simulink model "Phase1_Mark2"  (R2024b)
settings: Solver=ode23tb  StartTime=0.0  StopTime=inf  FixedStep=.001  RelTol=1e-1
model workspace (MAT data in the model file):
  A_mu = 10
  B_reff = 8.386
  CONVERTER_DATA = [0 0.1 0.2 0.3 0.4 0.5 0.6 0.7 0.8 0.81 0.82 0.83 ... (63 elements, 21x3)]
  Cps = 2
  Cz = 7766.25
  DOWN_TABLE = [0 0 0 0 0 0 5 5 7.5 7.5 15 15 ... (30 elements, 6x5)]
  DOWN_TH_BP = [0 5 40 50 90 100]
  D_reff = 0.25826
  EMAP = [-40 215 245 264 264 267 267 267 267 267 -44 117 ... (110 elements, 10x11)]
  F0z = [6086.4 4324.8]
  F_reff = 0.07394
  F_zmax = 10000
  F_zmin = 100
  F_zo = 4000
  Kz = 48000
  MF : object (value not decoded)
  NCyl = 6
  NE_VEC = [800 1200 1600 2000 2400 2800 3200 3600 4000 4400 4800]
  Pstd = 101325
  Rair = 287
  SUS : object (value not decoded)
  TH_VEC = [0; 20; 30; 40; 50; 60; 70; 80; 90; 100]
  TWAITdn = 1.25
  TWAITup = 0.1
  Tin = [1 2 3 4 5 6 7 8 9 10 2 2 ... (20 elements, 10x2)]
  Tstd = 293.15
  UP_TABLE = [7.5 7.5 15 25 40 40 25 25 35 45 70 80 ... (30 elements, 6x5)]
  UP_TH_BP = [0 25 35 50 90 100]
  VEH : object (value not decoded)
  V_o = 16.7
  V_xlow = 1
  Vd = 0.00346
  WH : object (value not decoded)
  a = 1.515
  alpha_max = 1.5
  alpha_min = -1.5
  b = 1.504
  c_zo = 209651
  epsilon = 0.1
  f_air = [0 0 0 0 0 0 0 0 0 0 0 0 ... (256 elements, 16x16)]
  f_co = [0 0 0 0 0 0 0 0 0 0 0 0 ... (256 elements, 16x16)]
  f_co2 = [0 0 0 0 0 0 0 0 0 0 0 0 ... (256 elements, 16x16)]
  f_eff = [352.135682859 352.135682859 320.724378192 303.655312657 295.930136708 291.240087194 291.240271258 291.240312459 291.240275452 291.240198499 291.240100781 291.240018769 ... (256 elements, 16x16)]
  f_fuel = [0 0 0 0 0 0 0 0 0 0 0 0 ... (256 elements, 16x16)]
  f_hc = [0 0 0 0 0 0 0 0 0 0 0 0 ... (256 elements, 16x16)]
  f_nox = [0 0 0 0 0 0 0 0 0 0 0 0 ... (256 elements, 16x16)]
  f_pm = [0 0 0 0 0 0 0 0 0 0 0 0 ... (256 elements, 16x16)]
  f_susp_axl_bp = [1 2]
  f_susp_dz_bp = [-4 -0.14 -0.13 -0.12 -0.11 -0.1 -0.09 -0.08 -0.07 -0.06 -0.05 -0.04 ... (31 elements, 1x31)]
  f_susp_dzdot_bp = [-4 -0.14 -0.13 -0.12 -0.11 -0.1 -0.09 -0.08 -0.07 -0.06 -0.05 -0.04 ... (31 elements, 1x31)]
  f_susp_fmz = [-213379.591456 -28099.591456 -27619.591456 -27139.591456 -26659.591456 -26179.591456 -25699.591456 -25219.591456 -24739.591456 -24259.591456 -23779.591456 -23299.591456 ... (468968 elements, 31x31x61x2x4)]
  f_susp_geom = [-0.832564012244 0.043269987756 0.045538987756 0.047807987756 0.050076987756 0.052345987756 0.054614987756 0.056883987756 0.059152987756 0.061421987756 0.063690987756 0.065959987756 ... (11346 elements, 31x61x2x3)]
  f_susp_strgdelta_bp = [-0.523598775598 -0.506145483078 -0.488692190558 -0.471238898038 -0.453785605519 -0.436332312999 -0.418879020479 -0.401425727959 -0.383972435439 -0.366519142919 -0.349065850399 -0.331612557879 ... (61 elements, 1x61)]
  f_tbrake = [0 76.8593923996 105.140482948 131.533638111 157.926793274 176.658631717 176.65727296 176.656856686 176.656879077 176.657093756 176.657404516 176.65772406 ... (256 elements, 16x16)]
  f_tbrake_n_bpt = [0 649.519052838 912.419621844 1175.32019085 1438.22075986 1701.12132886 1964.02189787 2226.92246687 2489.82303588 2752.72360489 3015.62417389 3278.5247429 ... (16 elements, 1x16)]
  f_tbrake_t_bpt = [0 34.6410161514 61.0341713143 87.4273264773 113.82048164 140.213636803 166.606791966 192.999947129 219.393102292 245.786257455 272.179412618 298.572567781 ... (16 elements, 1x16)]
  f_texh = [766.752464599 766.752464599 786.17542386 801.679939032 884.591982581 910.574397722 910.571871054 910.570774534 910.570601632 910.570821151 910.571247242 910.571639815 ... (256 elements, 16x16)]
  f_twc_eff_co = [0.17 0.25 0.45 0.99 0.99 0.99 0.99]
  f_twc_eff_hc = [0.21 0.375 0.75 0.98 0.98 0.98 0.98]
  f_twc_eff_lam = [0.909090909 0.944055944 0.979020979 1 1.013986014 1.048951049 1.083916084]
  f_twc_eff_nox = [0.98 0.98 0.98 0.97 0.05 0.02 0]
  h = 0.134
  k_z = 50
  kappa_max = 1.5
  kappa_min = -1.5
  lam_Cx = 1
  lam_Cy = 1
  lam_Cz = 1
  lam_Ex = 1
  lam_Ey = 1
  lam_F_zo = 1
  lam_Hx = 1
  lam_Hy = 1
  lam_Kxkappa = 1
  lam_Kyalpha = 1
  lam_Kygamma = 1
  lam_Kzgamma = 1
  lam_Mr = 1
  lam_Mx = 1
  lam_My = 1
  lam_S = 1
  lam_VMx = 1
  lam_Vx = 1
  lam_Vy = 1
  lam_Vykappa = 1
  lam_muV = 0
  lam_mux = 1
  lam_muy = 1
  lam_t = 1
  lam_xalpha = 1
  lam_ykappa = 1
  numWheel = 4
  p_Cx1 = 1.579
  p_Cy1 = 1.3332
  p_Dx1 = 1.0422
  p_Dx2 = -0.08285
  p_Dx3 = 0
  p_Dy1 = 0.8784
  p_Dy2 = -0.06445
  p_Dy3 = 0
  p_Ex1 = 0.11185
  p_Ex2 = 0.3127
  p_Ex3 = 0
  p_Ex4 = 0.001603
  p_Ey1 = -0.8227
  p_Ey2 = -0.6062
  p_Ey3 = 0.09825
  p_Ey4 = -6.546
  p_Ey5 = 0
  p_Fz1 = 0.7098
  p_Hx1 = 0.00021585
  p_Hx2 = 0.0011538
  p_Hy1 = -0.0018043
  p_Hy2 = 0.003518
  p_Kx1 = 21.69
  p_Kx2 = 13.774
  p_Kx3 = -0.4119
  p_Ky1 = -15.314
  p_Ky2 = 1.7044
  p_Ky3 = 0.36986
  p_Ky4 = 1.9896
  p_Ky5 = 0
  p_Ky6 = -0.9004
  p_Ky7 = -0.2328
  p_Vx1 = 1.5973e-05
  p_Vx2 = 0.0001043
  p_Vy1 = -0.006642
  p_Vy2 = 0.03597
  p_Vy3 = -0.1621
  p_Vy4 = -0.4908
  p_pmx1 = 0
  p_px1 = -0.3489
  p_px2 = 0.382
  p_px3 = -0.09634
  p_px4 = 0.06447
  p_py1 = -0.6249
  p_py2 = -0.06535
  p_py3 = -0.1668
  p_py4 = 0.2834
  p_py5 = 0
  path : object (value not decoded)
  pio = 220000
  q_Fcx = 0
  q_Fz2 = 15.4
  q_Fzy = 0
  q_reo = 0.9974
  q_sx1 = -0.007764
  q_sx10 = 0.2824
  q_sx11 = 5.349
  q_sx12 = 0
  q_sx13 = 0
  q_sx14 = 0
  q_sx2 = 1.1915
  q_sx3 = 0.013948
  q_sx4 = 4.912
  q_sx5 = 1.02
  q_sx6 = 22.83
  q_sx7 = 0.7104
  q_sx8 = -0.023393
  q_sx9 = 0.6581
  q_sy1 = 0.00702
  q_sy2 = 0
  q_sy3 = 0.001515
  q_sy4 = 8.514e-05
  q_sy5 = 0
  q_sy6 = 0
  q_sy7 = 0.9008
  q_sy8 = -0.4089
  q_v1 = 0.0007742
  q_v2 = 0.04667
  r_Bx1 = 12.531
  r_Bx2 = 9.532
  r_Bx3 = 0
  r_By1 = 10.615
  r_By2 = 7.705
  r_By3 = 3.433e-06
  r_By4 = 0
  r_Cx1 = 1.019
  r_Cy1 = 1.0585
  r_Ex1 = -0.4487
  r_Ex2 = -0.4726
  r_Ey1 = 0.3132
  r_Ey2 = 7.63e-06
  r_Hx1 = 0.0002374
  r_Hy1 = 0.011646
  r_Hy2 = 7.63e-06
  r_Vy1 = 0.05654
  r_Vy2 = 7.63e-06
  r_Vy3 = 0
  r_Vy4 = 99.9
  r_Vy5 = 2
  r_Vy6 = 15.814
  r_o = 0.3135
  reqTmaxT = [nan 0.285774810084 0.647179872268 nan nan nan nan nan nan nan nan nan ... (168 elements, 21x8)]
  vehSpd = [0 2.77777777778 5.55555555556 8.33333333333 11.1111111111 13.8888888889 16.6666666667 19.4444444444 22.2222222222 25 27.7777777778 30.5555555556 ... (21 elements, 1x21)]
  vehWidth = 2
  w = 1
symbols that are objects in the model workspace (value not decoded): VEH
undefined symbols (not defined in the file or in its folder): Fzz, Fzzdot, InertFrm, pFz, psi, vdyntiremask, x_o, zdotFz, zFz
(part 7 of 24)

== system Phase1_Mark2/Longitudinal Wheels 4DOF/Velocity and Vertical Load/Dual/Dual Fz ==
  In1 : Inport
  Add : Sum
  Bus Selector6 : BusSelector  OutputSignals=BdyFrm.Forces.Tires.FrntTires.Lft.Fz,BdyFrm.Forces.Tires.FrntTires.Rght.Fz,BdyFrm.Forces.Tires.RearTires.Lft.Fz,BdyFrm.Forces.Tires.RearTires.Rght.Fz
  Cont LPF : Subsystem  mask{wc=100*2*pi, AbsoluteTolerance=auto, aMode=2}
      mask prompts: wc "Cutoff frequency, wc [rad/s]"; AbsoluteTolerance "Simulink:blkprm_prompts:ContinuousStateAbsoluteTolerance"
      mask init:
      | [~]=autosharedicon('autolibutils',gcb,0);
      mask TypeOptions AbsoluteTolerance: Integrator1/AbsoluteTolerance
      mask DialogControl AbsoluteTolerance Prompt: Absolute tolerance:
      mask Display: fprintf('LPF')
  Saturation : Saturate  UpperLimit=10e3  LowerLimit=100  ZeroCross=off
  Unsprung Mass : Constant  Value=[0 0 80 80].*9.81
  Vector Concatenate : Concatenate  NumInputs=4
  Out1 : Outport  VectorParamsAs1DForOutWhenUnconnected=off
  wires:
  In1/1 -> Bus Selector6/1
  Saturation/1 -> Cont LPF/1(u)
  Cont LPF/1(y) -> Add/1
  Vector Concatenate/1 -> Saturation/1
  Bus Selector6/2 -> Vector Concatenate/2  "<Fz>"
  Bus Selector6/1 -> Vector Concatenate/1  "<Fz>"
  Bus Selector6/3 -> Vector Concatenate/3  "<Fz>"
  Bus Selector6/4 -> Vector Concatenate/4  "<Fz>"
  Add/1 -> Out1/1
  Unsprung Mass/1 -> Add/2

== system Phase1_Mark2/Longitudinal Wheels 4DOF/Velocity and Vertical Load/Dual/Dual V ==
  In1 : Inport
  Bus Selector1 : BusSelector  OutputSignals=BdyFrm.FrntAxl.Lft.Vel.xdot,BdyFrm.FrntAxl.Lft.Vel.ydot,BdyFrm.FrntAxl.Lft.Vel.zdot  OutputAsBus=on
  Bus Selector2 : BusSelector  OutputSignals=BdyFrm.FrntAxl.Rght.Vel.xdot,BdyFrm.FrntAxl.Rght.Vel.ydot,BdyFrm.FrntAxl.Rght.Vel.zdot  OutputAsBus=on
  Bus Selector4 : BusSelector  OutputSignals=BdyFrm.RearAxl.Lft.Vel.xdot,BdyFrm.RearAxl.Lft.Vel.ydot,BdyFrm.RearAxl.Lft.Vel.zdot  OutputAsBus=on
  Bus Selector5 : BusSelector  OutputSignals=BdyFrm.RearAxl.Rght.Vel.xdot,BdyFrm.RearAxl.Rght.Vel.ydot,BdyFrm.RearAxl.Rght.Vel.zdot  OutputAsBus=on
  Bus to Vector{5..8} (4 alike) : BusToVector
  Vector Concatenate2 : Concatenate  NumInputs=4  Mode=Multidimensional array  ConcatenateDimension=2
  Out1 : Outport  VectorParamsAs1DForOutWhenUnconnected=off
  wires:
  Bus to Vector6/1 -> Vector Concatenate2/2
  Bus Selector2/1 -> Bus to Vector6/1
  Bus to Vector8/1 -> Vector Concatenate2/4
  Bus Selector4/1 -> Bus to Vector7/1
  Bus to Vector5/1 -> Vector Concatenate2/1
  Bus Selector1/1 -> Bus to Vector5/1
  In1/1 -> Bus Selector1/1, Bus Selector2/1, Bus Selector4/1, Bus Selector5/1
  Bus Selector5/1 -> Bus to Vector8/1
  Bus to Vector7/1 -> Vector Concatenate2/3
  Vector Concatenate2/1 -> Out1/1

== system Phase1_Mark2/Vehicle Body 3DOF External Longitudinal Wheels/Bicycle/Vehicle Body 3DOF Single Track/Cy ==
  note: 1) Add Subsystem or Model blocks as valid variant choices.
      | 2) You cannot connect blocks at this level. At simulation, connectivity is automatically
      | determined, based on the active variant and port name matching.
  alpha_f : Inport
  alpha_r : Inport  Port=2
  Cy const : Subsystem  VariantControl=0
  Cy const dual : Subsystem  VariantControl=2
  Cy table : Subsystem  VariantControl=1
  Cy table dual : Subsystem  VariantControl=3
  Cy_f : Outport  VectorParamsAs1DForOutWhenUnconnected=off
  Cy_r : Outport  Port=2  VectorParamsAs1DForOutWhenUnconnected=off

== system Phase1_Mark2/Vehicle Body 3DOF External Longitudinal Wheels/Bicycle/Vehicle Body 3DOF Single Track/Drag ==
  wind : Inport
  y : Inport  Port=2
  Temp : Inport  Port=3  Unit=K
  Constant : Constant  Value=0
  Demux : Demux  Outputs=3
  Drag Force : Subsystem  mask{A=Af, beta_w=beta_w, Cd=Cd, Cs=Cs, Cl=Cl, Cpm=Cpm, Lcpm=a+b, Crm=beta_w.*0, Cym=Cym, R=287.058, Pabs=Pabs}
      mask prompts: A "Effective area, A [m^s2]:"; beta_w "Relative wind angle vector, beta_w [rad]:"; Cd "Longitudinal drag coefficient, Cd [-]:"; Cs "Side force coefficient data, Cs [-]:"; Cl "Lift coefficient, Cl [-]:"; Cpm "Pitch moment coefficient, Cpm [-]:"; Lcpm "Pitch moment length, Lcpm"; Crm "Roll moment coefficient data, Crm [-]:"; Cym "Yaw moment coefficient data, Cym [-]:"; R "Gas constant, R [J/(kg*K)]:"; Pabs "Absoulte pressure, Pabs [Pa]:"
  Selector2 : Selector  InputPortWidth=4  IndexOptions=Index vector (dialog)  Indices=[1:3]  OutputSizes=1
  Unary Minus : UnaryMinus
  Unary Minus1 : UnaryMinus
  Vector Concatenate1 : Concatenate  NumInputs=3
  inertial2body : Subsystem
  Fd : Outport  VectorParamsAs1DForOutWhenUnconnected=off
  Md : Outport  Port=2  VectorParamsAs1DForOutWhenUnconnected=off
  wires:
  Temp/1 -> Drag Force/3(T)
  inertial2body/1(Windxyz) -> Drag Force/2(Body Axis Wind)
  wind/1 -> inertial2body/2(WindXYZ)
  Demux/3 -> inertial2body/1(psi)
  Demux/1 -> Vector Concatenate1/1
  Demux/2 -> Vector Concatenate1/2
  Constant/1 -> Vector Concatenate1/3
  Vector Concatenate1/1 -> Drag Force/1(Body Axis Vel)
  Selector2/1 -> Demux/1
  Drag Force/2(Md) -> Unary Minus1/1
  y/1 -> Selector2/1
  Drag Force/1(Fd) -> Unary Minus/1
  Unary Minus/1 -> Fd/1
  Unary Minus1/1 -> Md/1

== system Phase1_Mark2/Vehicle Body 3DOF External Longitudinal Wheels/Bicycle/Vehicle Body 3DOF Single Track/Signal Routing ==
  note: 1) Add Subsystem or Model blocks as valid variant choices.
      | 2) You cannot connect blocks at this level. At simulation, connectivity is automatically
      | determined, based on the active variant and port name matching.
  y : Inport
  Fbody : Inport  Port=2  Unit=N
  MTotal : Inport  Port=3  Unit=N*m
  FOut : Inport  Port=4
  FTire : Inport  Port=5  Unit=N
  Fg : Inport  Port=6  Unit=N
  FDrag : Inport  Port=7  Unit=N
  MDrag : Inport  Port=8  Unit=N*m
  FExt : Inport  Port=9  Unit=N
  MExt : Inport  Port=10  Unit=N*m
  x : Inport  Port=11
  WhlAngF : Inport  Port=12
  WhlAngR : Inport  Port=13
  Fh : Inport  Port=14  Unit=N
  Mh : Inport  Port=15  Unit=N*m
  Xo : Inport  Port=16
  Signal Routing : Subsystem  VariantControl=0
  Signal Routing Dual : Subsystem  VariantControl=1
  Info : Outport  VectorParamsAs1DForOutWhenUnconnected=off
  xdot : Outport  Port=2  VectorParamsAs1DForOutWhenUnconnected=off
  ydot : Outport  Port=3  VectorParamsAs1DForOutWhenUnconnected=off
  psi : Outport  Port=4  VectorParamsAs1DForOutWhenUnconnected=off
  r : Outport  Port=5  VectorParamsAs1DForOutWhenUnconnected=off
  FzF : Outport  Port=6  VectorParamsAs1DForOutWhenUnconnected=off
  FzR : Outport  Port=7  VectorParamsAs1DForOutWhenUnconnected=off

== system Phase1_Mark2/Vehicle Body 3DOF External Longitudinal Wheels/Bicycle/Vehicle Body 3DOF Single Track/friction ==
  note: 1) Add Subsystem or Model blocks as valid variant choices.
      | 2) You cannot connect blocks at this level. At simulation, connectivity is automatically
      | determined, based on the active variant and port name matching.
  mu_in : Inport  Unit=1
  mu ext : Subsystem  VariantControl=1
  mu ext dual : Subsystem  VariantControl=3
  mu int : Subsystem  VariantControl=0
  mu int dual : Subsystem  VariantControl=2
  mu_out : Outport  Unit=1  VectorParamsAs1DForOutWhenUnconnected=off

== system Phase1_Mark2/Vehicle Body 3DOF External Longitudinal Wheels/Bicycle/Vehicle Body 3DOF Single Track/front forces ==
  note: 1) Add Subsystem or Model blocks as valid variant choices.
      | 2) You cannot connect blocks at this level. At simulation, connectivity is automatically
      | determined, based on the active variant and port name matching.
  F_in : Inport  Unit=N
  ext : Subsystem  VariantControl=2
  ext dual : Subsystem  VariantControl=5
  ext long : Subsystem  VariantControl=1
  ext long dual : Subsystem  VariantControl=4
  int : Subsystem  VariantControl=0
  int dual : Subsystem  VariantControl=3
  F_out : Outport  Unit=N  VectorParamsAs1DForOutWhenUnconnected=off

== system Phase1_Mark2/Vehicle Body 3DOF External Longitudinal Wheels/Bicycle/Vehicle Body 3DOF Single Track/front steer ==
  note: 1) Add Subsystem or Model blocks as valid variant choices.
      | 2) You cannot connect blocks at this level. At simulation, connectivity is automatically
      | determined, based on the active variant and port name matching.
  delta_in : Inport  Unit=rad
  delta ext : Subsystem  VariantControl=1
  delta ext dual : Subsystem  VariantControl=3
  delta int : Subsystem  VariantControl=0
  delta int dual : Subsystem  VariantControl=2
  delta_out : Outport  Unit=rad  VectorParamsAs1DForOutWhenUnconnected=off

== system Phase1_Mark2/Vehicle Body 3DOF External Longitudinal Wheels/Bicycle/Vehicle Body 3DOF Single Track/hitch geometry parameters ==
  note: 1) Add Subsystem or Model blocks as valid variant choices.
      | 2) You cannot connect blocks at this level. At simulation, connectivity is automatically
      | determined, based on the active variant and port name matching.
  hitch active bicycle : Subsystem  VariantControl=1
  hitch active dual track : Subsystem  VariantControl=2
  hitch inactive : Subsystem  VariantControl=3
  dh_out : Outport  Unit=m  VectorParamsAs1DForOutWhenUnconnected=off
  hl_out : Outport  Port=2  Unit=m  VectorParamsAs1DForOutWhenUnconnected=off
  hh_out : Outport  Port=3  Unit=m  VectorParamsAs1DForOutWhenUnconnected=off

== system Phase1_Mark2/Vehicle Body 3DOF External Longitudinal Wheels/Bicycle/Vehicle Body 3DOF Single Track/rear forces ==
  note: 1) Add Subsystem or Model blocks as valid variant choices.
      | 2) You cannot connect blocks at this level. At simulation, connectivity is automatically
      | determined, based on the active variant and port name matching.
  F_in : Inport  Unit=N
  ext : Subsystem  VariantControl=2
  ext dual : Subsystem  VariantControl=5
  ext long : Subsystem  VariantControl=1
  ext long dual : Subsystem  VariantControl=4
  int : Subsystem  VariantControl=0
  int dual : Subsystem  VariantControl=3
  F_out : Outport  Unit=N  VectorParamsAs1DForOutWhenUnconnected=off

== system Phase1_Mark2/Vehicle Body 3DOF External Longitudinal Wheels/Bicycle/Vehicle Body 3DOF Single Track/rear steer ==
  note: 1) Add Subsystem or Model blocks as valid variant choices.
      | 2) You cannot connect blocks at this level. At simulation, connectivity is automatically
      | determined, based on the active variant and port name matching.
  delta_in : Inport  Unit=rad
  delta ext : Subsystem  VariantControl=1
  delta ext dual : Subsystem  VariantControl=3
  delta int : Subsystem  VariantControl=0
  delta int dual : Subsystem  VariantControl=2
  delta_out : Outport  Unit=rad  VectorParamsAs1DForOutWhenUnconnected=off

== system Phase1_Mark2/Vehicle Body 3DOF External Longitudinal Wheels/Bicycle/Vehicle Body 3DOF Single Track/sigma ==
  note: 1) Add Subsystem or Model blocks as valid variant choices.
      | 2) You cannot connect blocks at this level. At simulation, connectivity is automatically
      | determined, based on the active variant and port name matching.
  y : Inport
  no sigma : Subsystem  VariantControl=0
  no sigma dual : Subsystem  VariantControl=2
  sigma : Subsystem  VariantControl=1
  sigma dual : Subsystem  VariantControl=3
  alpha_f : Outport  VectorParamsAs1DForOutWhenUnconnected=off
  alpha_r : Outport  Port=2  VectorParamsAs1DForOutWhenUnconnected=off

== system Phase1_Mark2/Vehicle Body 3DOF External Longitudinal Wheels/Bicycle/Vehicle Body 3DOF Single Track/state ==
  note: 1) Add Subsystem or Model blocks as valid variant choices.
      | 2) You cannot connect blocks at this level. At simulation, connectivity is automatically
      | determined, based on the active variant and port name matching.
  xdot : Inport  Unit=m/s
  xddot_in : Inport  Port=2  PortDimensions=4
  extState : Inport  Port=3
  xdot ext : Subsystem  VariantControl=1
  xdot int : Subsystem  VariantControl=0
  xddot_out : Outport  VectorParamsAs1DForOutWhenUnconnected=off

== system Phase1_Mark2/Vehicle Body 3DOF External Longitudinal Wheels/Bicycle/Vehicle Body 3DOF Single Track/wind ==
  note: 1) Add Subsystem or Model blocks as valid variant choices.
      | 2) You cannot connect blocks at this level. At simulation, connectivity is automatically
      | determined, based on the active variant and port name matching.
  wind_in : Inport  Unit=m/s
  wind ext : Subsystem  VariantControl=1
  wind int : Subsystem  VariantControl=0
  wind_out : Outport  Unit=m/s  VectorParamsAs1DForOutWhenUnconnected=off

== system Phase1_Mark2/Vehicle Body 3DOF External Longitudinal Wheels/Dual/Vehicle Body 3DOF Dual Track/Cy ==
  note: 1) Add Subsystem or Model blocks as valid variant choices.
      | 2) You cannot connect blocks at this level. At simulation, connectivity is automatically
      | determined, based on the active variant and port name matching.
  alpha_f : Inport
  alpha_r : Inport  Port=2
  Cy const : Subsystem  VariantControl=0
  Cy const dual : Subsystem  VariantControl=2
  Cy table : Subsystem  VariantControl=1
  Cy table dual : Subsystem  VariantControl=3
  Cy_f : Outport  VectorParamsAs1DForOutWhenUnconnected=off
  Cy_r : Outport  Port=2  VectorParamsAs1DForOutWhenUnconnected=off

== system Phase1_Mark2/Vehicle Body 3DOF External Longitudinal Wheels/Dual/Vehicle Body 3DOF Dual Track/Drag ==
  wind : Inport
  y : Inport  Port=2
  Temp : Inport  Port=3  Unit=K
  Constant : Constant  Value=0
  Demux : Demux  Outputs=3
  Drag Force : Subsystem  mask{A=Af, beta_w=beta_w, Cd=Cd, Cs=Cs, Cl=Cl, Cpm=Cpm, Lcpm=a+b, Crm=beta_w.*0, Cym=Cym, R=287.058, Pabs=Pabs}
      mask prompts: A "Effective area, A [m^s2]:"; beta_w "Relative wind angle vector, beta_w [rad]:"; Cd "Longitudinal drag coefficient, Cd [-]:"; Cs "Side force coefficient data, Cs [-]:"; Cl "Lift coefficient, Cl [-]:"; Cpm "Pitch moment coefficient, Cpm [-]:"; Lcpm "Pitch moment length, Lcpm"; Crm "Roll moment coefficient data, Crm [-]:"; Cym "Yaw moment coefficient data, Cym [-]:"; R "Gas constant, R [J/(kg*K)]:"; Pabs "Absoulte pressure, Pabs [Pa]:"
  Selector2 : Selector  InputPortWidth=4  IndexOptions=Index vector (dialog)  Indices=[1:3]  OutputSizes=1
  Unary Minus : UnaryMinus
  Unary Minus1 : UnaryMinus
  Vector Concatenate1 : Concatenate  NumInputs=3
  inertial2body : Subsystem
  Fd : Outport  VectorParamsAs1DForOutWhenUnconnected=off
  Md : Outport  Port=2  VectorParamsAs1DForOutWhenUnconnected=off
  wires:
  Temp/1 -> Drag Force/3(T)
  inertial2body/1(Windxyz) -> Drag Force/2(Body Axis Wind)
  wind/1 -> inertial2body/2(WindXYZ)
  Demux/3 -> inertial2body/1(psi)
  Demux/1 -> Vector Concatenate1/1
  Demux/2 -> Vector Concatenate1/2
  Constant/1 -> Vector Concatenate1/3
  Vector Concatenate1/1 -> Drag Force/1(Body Axis Vel)
  Selector2/1 -> Demux/1
  Drag Force/2(Md) -> Unary Minus1/1
  y/1 -> Selector2/1
  Drag Force/1(Fd) -> Unary Minus/1
  Unary Minus/1 -> Fd/1
  Unary Minus1/1 -> Md/1

== system Phase1_Mark2/Vehicle Body 3DOF External Longitudinal Wheels/Dual/Vehicle Body 3DOF Dual Track/Signal Routing ==
  note: 1) Add Subsystem or Model blocks as valid variant choices.
      | 2) You cannot connect blocks at this level. At simulation, connectivity is automatically
      | determined, based on the active variant and port name matching.
  y : Inport
  Fbody : Inport  Port=2  Unit=N
  MTotal : Inport  Port=3  Unit=N*m
  FOut : Inport  Port=4
  FTire : Inport  Port=5  Unit=N
  Fg : Inport  Port=6  Unit=N
  FDrag : Inport  Port=7  Unit=N
  MDrag : Inport  Port=8  Unit=N*m
  FExt : Inport  Port=9  Unit=N
  MExt : Inport  Port=10  Unit=N*m
  x : Inport  Port=11
  WhlAngF : Inport  Port=12
  WhlAngR : Inport  Port=13
  Fh : Inport  Port=14  Unit=N
  Mh : Inport  Port=15  Unit=N*m
  Xo : Inport  Port=16
  Signal Routing : Subsystem  VariantControl=0
  Signal Routing Dual : Subsystem  VariantControl=1
  Info : Outport  VectorParamsAs1DForOutWhenUnconnected=off
  xdot : Outport  Port=2  VectorParamsAs1DForOutWhenUnconnected=off
  ydot : Outport  Port=3  VectorParamsAs1DForOutWhenUnconnected=off
  psi : Outport  Port=4  VectorParamsAs1DForOutWhenUnconnected=off
  r : Outport  Port=5  VectorParamsAs1DForOutWhenUnconnected=off
  FzF : Outport  Port=6  VectorParamsAs1DForOutWhenUnconnected=off
  FzR : Outport  Port=7  VectorParamsAs1DForOutWhenUnconnected=off

== system Phase1_Mark2/Vehicle Body 3DOF External Longitudinal Wheels/Dual/Vehicle Body 3DOF Dual Track/friction ==
  note: 1) Add Subsystem or Model blocks as valid variant choices.
      | 2) You cannot connect blocks at this level. At simulation, connectivity is automatically
      | determined, based on the active variant and port name matching.
  mu_in : Inport  Unit=1
  mu ext : Subsystem  VariantControl=1
  mu ext dual : Subsystem  VariantControl=3
  mu int : Subsystem  VariantControl=0
  mu int dual : Subsystem  VariantControl=2
  mu_out : Outport  Unit=1  VectorParamsAs1DForOutWhenUnconnected=off

== system Phase1_Mark2/Vehicle Body 3DOF External Longitudinal Wheels/Dual/Vehicle Body 3DOF Dual Track/front forces ==
  note: 1) Add Subsystem or Model blocks as valid variant choices.
      | 2) You cannot connect blocks at this level. At simulation, connectivity is automatically
      | determined, based on the active variant and port name matching.
  F_in : Inport  Unit=N
  ext : Subsystem  VariantControl=2
  ext dual : Subsystem  VariantControl=5
  ext long : Subsystem  VariantControl=1
  ext long dual : Subsystem  VariantControl=4
  int : Subsystem  VariantControl=0
  int dual : Subsystem  VariantControl=3
  F_out : Outport  Unit=N  VectorParamsAs1DForOutWhenUnconnected=off

== system Phase1_Mark2/Vehicle Body 3DOF External Longitudinal Wheels/Dual/Vehicle Body 3DOF Dual Track/front steer ==
  note: 1) Add Subsystem or Model blocks as valid variant choices.
      | 2) You cannot connect blocks at this level. At simulation, connectivity is automatically
      | determined, based on the active variant and port name matching.
  delta_in : Inport  Unit=rad
  delta ext : Subsystem  VariantControl=1
  delta ext dual : Subsystem  VariantControl=3
  delta int : Subsystem  VariantControl=0
  delta int dual : Subsystem  VariantControl=2
  delta_out : Outport  Unit=rad  VectorParamsAs1DForOutWhenUnconnected=off

== system Phase1_Mark2/Vehicle Body 3DOF External Longitudinal Wheels/Dual/Vehicle Body 3DOF Dual Track/hitch geometry parameters ==
  note: 1) Add Subsystem or Model blocks as valid variant choices.
      | 2) You cannot connect blocks at this level. At simulation, connectivity is automatically
      | determined, based on the active variant and port name matching.
  hitch active bicycle : Subsystem  VariantControl=1
  hitch active dual track : Subsystem  VariantControl=2
  hitch inactive : Subsystem  VariantControl=3
  dh_out : Outport  Unit=m  VectorParamsAs1DForOutWhenUnconnected=off
  hl_out : Outport  Port=2  Unit=m  VectorParamsAs1DForOutWhenUnconnected=off
  hh_out : Outport  Port=3  Unit=m  VectorParamsAs1DForOutWhenUnconnected=off

== system Phase1_Mark2/Vehicle Body 3DOF External Longitudinal Wheels/Dual/Vehicle Body 3DOF Dual Track/rear forces ==
  note: 1) Add Subsystem or Model blocks as valid variant choices.
      | 2) You cannot connect blocks at this level. At simulation, connectivity is automatically
      | determined, based on the active variant and port name matching.
  F_in : Inport  Unit=N
  ext : Subsystem  VariantControl=2
  ext dual : Subsystem  VariantControl=5
  ext long : Subsystem  VariantControl=1
  ext long dual : Subsystem  VariantControl=4
  int : Subsystem  VariantControl=0
  int dual : Subsystem  VariantControl=3
  F_out : Outport  Unit=N  VectorParamsAs1DForOutWhenUnconnected=off

== system Phase1_Mark2/Vehicle Body 3DOF External Longitudinal Wheels/Dual/Vehicle Body 3DOF Dual Track/rear steer ==
  note: 1) Add Subsystem or Model blocks as valid variant choices.
      | 2) You cannot connect blocks at this level. At simulation, connectivity is automatically
      | determined, based on the active variant and port name matching.
  delta_in : Inport  Unit=rad
  delta ext : Subsystem  VariantControl=1
  delta ext dual : Subsystem  VariantControl=3
  delta int : Subsystem  VariantControl=0
  delta int dual : Subsystem  VariantControl=2
  delta_out : Outport  Unit=rad  VectorParamsAs1DForOutWhenUnconnected=off

== system Phase1_Mark2/Vehicle Body 3DOF External Longitudinal Wheels/Dual/Vehicle Body 3DOF Dual Track/sigma ==
  note: 1) Add Subsystem or Model blocks as valid variant choices.
      | 2) You cannot connect blocks at this level. At simulation, connectivity is automatically
      | determined, based on the active variant and port name matching.
  y : Inport
  no sigma : Subsystem  VariantControl=0
  no sigma dual : Subsystem  VariantControl=2
  sigma : Subsystem  VariantControl=1
  sigma dual : Subsystem  VariantControl=3
  alpha_f : Outport  VectorParamsAs1DForOutWhenUnconnected=off
  alpha_r : Outport  Port=2  VectorParamsAs1DForOutWhenUnconnected=off

== system Phase1_Mark2/Vehicle Body 3DOF External Longitudinal Wheels/Dual/Vehicle Body 3DOF Dual Track/state ==
  note: 1) Add Subsystem or Model blocks as valid variant choices.
      | 2) You cannot connect blocks at this level. At simulation, connectivity is automatically
      | determined, based on the active variant and port name matching.
  xdot : Inport  Unit=m/s
  xddot_in : Inport  Port=2  PortDimensions=4
  extState : Inport  Port=3
  xdot ext : Subsystem  VariantControl=1
  xdot int : Subsystem  VariantControl=0
  xddot_out : Outport  VectorParamsAs1DForOutWhenUnconnected=off

== system Phase1_Mark2/Vehicle Body 3DOF External Longitudinal Wheels/Dual/Vehicle Body 3DOF Dual Track/wind ==
  note: 1) Add Subsystem or Model blocks as valid variant choices.
      | 2) You cannot connect blocks at this level. At simulation, connectivity is automatically
      | determined, based on the active variant and port name matching.
  wind_in : Inport  Unit=m/s
  wind ext : Subsystem  VariantControl=1
  wind int : Subsystem  VariantControl=0
  wind_out : Outport  Unit=m/s  VectorParamsAs1DForOutWhenUnconnected=off

== system Phase1_Mark2/Longitudinal Wheels 4DOF/Axle Forces/Bicycle/Wheel to Body Transform/Rotation Angles to Direction Cosine Matrix ==
  In1 : Inport  Unit=rad  PortDimensions=3
  Create 3x3 Matrix : Subsystem  mask(Create 3x3 Matrix){aMode=aMode}
      mask help: shared_aeroblks:sharedaeroblkutil:blockCreate3x3MatrixDesc
      mask init:
      | if aerosharedtest(gcb)
      |     aerosharedicon('shared');
      | else
      |     sharedautoicon('shared');
      | end
      mask Help: eval('if license(''test'',''Aerospace_Blockset'')aerosharedhelp(''create_threebythree_matrix'');elseif license(''test'',''Powertrain_Blockset'')sharedautohelp(''create_threebythree_matrix'');end')
      mask Display:
      | port_label('input',1,'A_{11}','texmode','on');
      | port_label('input',2,'A_{12}','texmode','on');
      | port_label('input',3,'A_{13}','texmode','on');
      | port_label('input',4,'A_{21}','texmode','on');
      | port_label('input',5,'A_{22}','texmode','on');
      | port_label('input',6,'A_{23}','texmode','on');
      | port_label('input',7,'A_{31}','texmode','on');
      | port_label('input',8,'A_{32}','texmode','on');
      | port_label('input',9,'A_{33}','texmode','on');
      | port_label('output',1,'A','texmode','on');
  Fcn11 : Fcn  Expr=u(5)*u(4)
  Fcn12 : Fcn  Expr=u(5)*u(1)
  Fcn13 : Fcn  Expr=-u(2)
  Fcn21 : Fcn  Expr=u(3)*u(2)*u(4) - u(6)*u(1)
  Fcn22 : Fcn  Expr=u(3)*u(2)*u(1) + u(6)*u(4)
  Fcn23 : Fcn  Expr=u(3)*u(5)
  Fcn31 : Fcn  Expr=u(6)*u(2)*u(4) + u(3)*u(1)
  Fcn32 : Fcn  Expr=u(6)*u(2)*u(1) - u(3)*u(4)
  Fcn33 : Fcn  Expr=u(6)*u(5)
  Mux : Mux  Inputs=2
  sincos : Trigonometry  Operator=sincos
  Out1 : Outport  Unit=1  PortDimensions=[3,3]  VectorParamsAs1DForOutWhenUnconnected=off
  wires:
  In1/1 -> sincos/1
  Create 3x3 Matrix/1(Matrix) -> Out1/1
  sincos/1 -> Mux/1
  sincos/2 -> Mux/2
  Mux/1 -> Fcn11/1, Fcn12/1, Fcn13/1, Fcn21/1, Fcn32/1, Fcn33/1, Fcn31/1, Fcn23/1, Fcn22/1
  Fcn11/1 -> Create 3x3 Matrix/1(M11)
  Fcn12/1 -> Create 3x3 Matrix/2(M12)
  Fcn13/1 -> Create 3x3 Matrix/3(M13)
  Fcn21/1 -> Create 3x3 Matrix/4(M21)
  Fcn31/1 -> Create 3x3 Matrix/7(M31)
  Fcn22/1 -> Create 3x3 Matrix/5(M22)
  Fcn23/1 -> Create 3x3 Matrix/6(M23)
  Fcn32/1 -> Create 3x3 Matrix/8(M32)
  Fcn33/1 -> Create 3x3 Matrix/9(M33)

== system Phase1_Mark2/Longitudinal Wheels 4DOF/Axle Forces/Bicycle/Wheel to Body Transform/Rotation Angles to Direction Cosine Matrix1 ==
  In1 : Inport  Unit=rad  PortDimensions=3
  Create 3x3 Matrix : Subsystem  mask(Create 3x3 Matrix){aMode=aMode}
      mask help: shared_aeroblks:sharedaeroblkutil:blockCreate3x3MatrixDesc
      mask init:
      | if aerosharedtest(gcb)
      |     aerosharedicon('shared');
      | else
      |     sharedautoicon('shared');
      | end
      mask Help: eval('if license(''test'',''Aerospace_Blockset'')aerosharedhelp(''create_threebythree_matrix'');elseif license(''test'',''Powertrain_Blockset'')sharedautohelp(''create_threebythree_matrix'');end')
      mask Display:
      | port_label('input',1,'A_{11}','texmode','on');
      | port_label('input',2,'A_{12}','texmode','on');
      | port_label('input',3,'A_{13}','texmode','on');
      | port_label('input',4,'A_{21}','texmode','on');
      | port_label('input',5,'A_{22}','texmode','on');
      | port_label('input',6,'A_{23}','texmode','on');
      | port_label('input',7,'A_{31}','texmode','on');
      | port_label('input',8,'A_{32}','texmode','on');
      | port_label('input',9,'A_{33}','texmode','on');
      | port_label('output',1,'A','texmode','on');
  Fcn11 : Fcn  Expr=u(5)*u(4)
  Fcn12 : Fcn  Expr=u(5)*u(1)
  Fcn13 : Fcn  Expr=-u(2)
  Fcn21 : Fcn  Expr=u(3)*u(2)*u(4) - u(6)*u(1)
  Fcn22 : Fcn  Expr=u(3)*u(2)*u(1) + u(6)*u(4)
  Fcn23 : Fcn  Expr=u(3)*u(5)
  Fcn31 : Fcn  Expr=u(6)*u(2)*u(4) + u(3)*u(1)
  Fcn32 : Fcn  Expr=u(6)*u(2)*u(1) - u(3)*u(4)
  Fcn33 : Fcn  Expr=u(6)*u(5)
  Mux : Mux  Inputs=2
  sincos : Trigonometry  Operator=sincos
  Out1 : Outport  Unit=1  PortDimensions=[3,3]  VectorParamsAs1DForOutWhenUnconnected=off
  wires:
  In1/1 -> sincos/1
  Create 3x3 Matrix/1(Matrix) -> Out1/1
  sincos/1 -> Mux/1
  sincos/2 -> Mux/2
  Mux/1 -> Fcn11/1, Fcn12/1, Fcn13/1, Fcn21/1, Fcn32/1, Fcn33/1, Fcn31/1, Fcn23/1, Fcn22/1
  Fcn11/1 -> Create 3x3 Matrix/1(M11)
  Fcn12/1 -> Create 3x3 Matrix/2(M12)
  Fcn13/1 -> Create 3x3 Matrix/3(M13)
  Fcn21/1 -> Create 3x3 Matrix/4(M21)
  Fcn31/1 -> Create 3x3 Matrix/7(M31)
  Fcn22/1 -> Create 3x3 Matrix/5(M22)
  Fcn23/1 -> Create 3x3 Matrix/6(M23)
  Fcn32/1 -> Create 3x3 Matrix/8(M32)
  Fcn33/1 -> Create 3x3 Matrix/9(M33)

== system Phase1_Mark2/Longitudinal Wheels 4DOF/Axle Forces/Dual/Wheel to Body Transform/Rotation Angles to Direction Cosine Matrix ==
  In1 : Inport  Unit=rad  PortDimensions=3
  Create 3x3 Matrix : Subsystem  mask(Create 3x3 Matrix){aMode=aMode}
      mask help: shared_aeroblks:sharedaeroblkutil:blockCreate3x3MatrixDesc
      mask init:
      | if aerosharedtest(gcb)
      |     aerosharedicon('shared');
      | else
      |     sharedautoicon('shared');
      | end
      mask Help: eval('if license(''test'',''Aerospace_Blockset'')aerosharedhelp(''create_threebythree_matrix'');elseif license(''test'',''Powertrain_Blockset'')sharedautohelp(''create_threebythree_matrix'');end')
      mask Display:
      | port_label('input',1,'A_{11}','texmode','on');
      | port_label('input',2,'A_{12}','texmode','on');
      | port_label('input',3,'A_{13}','texmode','on');
      | port_label('input',4,'A_{21}','texmode','on');
      | port_label('input',5,'A_{22}','texmode','on');
      | port_label('input',6,'A_{23}','texmode','on');
      | port_label('input',7,'A_{31}','texmode','on');
      | port_label('input',8,'A_{32}','texmode','on');
      | port_label('input',9,'A_{33}','texmode','on');
      | port_label('output',1,'A','texmode','on');
  Fcn11 : Fcn  Expr=u(5)*u(4)
  Fcn12 : Fcn  Expr=u(5)*u(1)
  Fcn13 : Fcn  Expr=-u(2)
  Fcn21 : Fcn  Expr=u(3)*u(2)*u(4) - u(6)*u(1)
  Fcn22 : Fcn  Expr=u(3)*u(2)*u(1) + u(6)*u(4)
  Fcn23 : Fcn  Expr=u(3)*u(5)
  Fcn31 : Fcn  Expr=u(6)*u(2)*u(4) + u(3)*u(1)
  Fcn32 : Fcn  Expr=u(6)*u(2)*u(1) - u(3)*u(4)
  Fcn33 : Fcn  Expr=u(6)*u(5)
  Mux : Mux  Inputs=2
  sincos : Trigonometry  Operator=sincos
  Out1 : Outport  Unit=1  PortDimensions=[3,3]  VectorParamsAs1DForOutWhenUnconnected=off
  wires:
  In1/1 -> sincos/1
  Create 3x3 Matrix/1(Matrix) -> Out1/1
  sincos/1 -> Mux/1
  sincos/2 -> Mux/2
  Mux/1 -> Fcn11/1, Fcn12/1, Fcn13/1, Fcn21/1, Fcn32/1, Fcn33/1, Fcn31/1, Fcn23/1, Fcn22/1
  Fcn11/1 -> Create 3x3 Matrix/1(M11)
  Fcn12/1 -> Create 3x3 Matrix/2(M12)
  Fcn13/1 -> Create 3x3 Matrix/3(M13)
  Fcn21/1 -> Create 3x3 Matrix/4(M21)
  Fcn31/1 -> Create 3x3 Matrix/7(M31)
  Fcn22/1 -> Create 3x3 Matrix/5(M22)
  Fcn23/1 -> Create 3x3 Matrix/6(M23)
  Fcn32/1 -> Create 3x3 Matrix/8(M32)
  Fcn33/1 -> Create 3x3 Matrix/9(M33)

== system Phase1_Mark2/Longitudinal Wheels 4DOF/Axle Forces/Dual/Wheel to Body Transform/Rotation Angles to Direction Cosine Matrix1 ==
  In1 : Inport  Unit=rad  PortDimensions=3
  Create 3x3 Matrix : Subsystem  mask(Create 3x3 Matrix){aMode=aMode}
      mask help: shared_aeroblks:sharedaeroblkutil:blockCreate3x3MatrixDesc
      mask init:
      | if aerosharedtest(gcb)
      |     aerosharedicon('shared');
      | else
      |     sharedautoicon('shared');
      | end
      mask Help: eval('if license(''test'',''Aerospace_Blockset'')aerosharedhelp(''create_threebythree_matrix'');elseif license(''test'',''Powertrain_Blockset'')sharedautohelp(''create_threebythree_matrix'');end')
      mask Display:
      | port_label('input',1,'A_{11}','texmode','on');
      | port_label('input',2,'A_{12}','texmode','on');
      | port_label('input',3,'A_{13}','texmode','on');
      | port_label('input',4,'A_{21}','texmode','on');
      | port_label('input',5,'A_{22}','texmode','on');
      | port_label('input',6,'A_{23}','texmode','on');
      | port_label('input',7,'A_{31}','texmode','on');
      | port_label('input',8,'A_{32}','texmode','on');
      | port_label('input',9,'A_{33}','texmode','on');
      | port_label('output',1,'A','texmode','on');
  Fcn11 : Fcn  Expr=u(5)*u(4)
  Fcn12 : Fcn  Expr=u(5)*u(1)
  Fcn13 : Fcn  Expr=-u(2)
  Fcn21 : Fcn  Expr=u(3)*u(2)*u(4) - u(6)*u(1)
  Fcn22 : Fcn  Expr=u(3)*u(2)*u(1) + u(6)*u(4)
  Fcn23 : Fcn  Expr=u(3)*u(5)
  Fcn31 : Fcn  Expr=u(6)*u(2)*u(4) + u(3)*u(1)
  Fcn32 : Fcn  Expr=u(6)*u(2)*u(1) - u(3)*u(4)
  Fcn33 : Fcn  Expr=u(6)*u(5)
  Mux : Mux  Inputs=2
  sincos : Trigonometry  Operator=sincos
  Out1 : Outport  Unit=1  PortDimensions=[3,3]  VectorParamsAs1DForOutWhenUnconnected=off
  wires:
  In1/1 -> sincos/1
  Create 3x3 Matrix/1(Matrix) -> Out1/1
  sincos/1 -> Mux/1
  sincos/2 -> Mux/2
  Mux/1 -> Fcn11/1, Fcn12/1, Fcn13/1, Fcn21/1, Fcn32/1, Fcn33/1, Fcn31/1, Fcn23/1, Fcn22/1
  Fcn11/1 -> Create 3x3 Matrix/1(M11)
  Fcn12/1 -> Create 3x3 Matrix/2(M12)
  Fcn13/1 -> Create 3x3 Matrix/3(M13)
  Fcn21/1 -> Create 3x3 Matrix/4(M21)
  Fcn31/1 -> Create 3x3 Matrix/7(M31)
  Fcn22/1 -> Create 3x3 Matrix/5(M22)
  Fcn23/1 -> Create 3x3 Matrix/6(M23)
  Fcn32/1 -> Create 3x3 Matrix/8(M32)
  Fcn33/1 -> Create 3x3 Matrix/9(M33)

== system Phase1_Mark2/Longitudinal Wheels 4DOF/Tires/Fiala/Fiala Tire/Bus Routing ==
  BrkPrs : Inport
  BrkTrq : Inport  Port=2
  omega : Inport  Port=3
  FLong : Inport  Port=4
  Flat : Inport  Port=5
  MOver : Inport  Port=6
  MRoll : Inport  Port=7
  MAlign : Inport  Port=8
  Re : Inport  Port=9
  Kappa : Inport  Port=10
  Alpha : Inport  Port=11
  a : Inport  Port=12
  b : Inport  Port=13
  z : Inport  Port=14
  zdot : Inport  Port=15
  GndFz : Inport  Port=16
  AxlTrq : Inport  Port=17
  Vx : Inport  Port=18
  Vy : Inport  Port=19
  Gamma : Inport  Port=20
  psidot : Inport  Port=21
  Prs : Inport  Port=22
  Gnd : Inport  Port=23
  Fext : Inport  Port=24
  WhlTrq : Inport  Port=25
  RL : Inport  Port=26
  RadialDeflct : Inport  Port=27
  Bus Creator : BusCreator  Inputs=27
  Signal Specification{,3,7,9..10,22..23} (7 alike) : SignalSpecification  Unit=m
  Signal Specification1 : SignalSpecification  Unit=1
  Signal Specification{5,8,15..17} (5 alike) : SignalSpecification  Unit=N*m
  Signal Specification{6,18..20} (4 alike) : SignalSpecification  Unit=N
  Signal Specification2 : SignalSpecification  Unit=rad
  Signal Specification21 : SignalSpecification  Unit=rad/s
  Signal Specification4 : SignalSpecification  Unit=m/s
  Info : Outport  VectorParamsAs1DForOutWhenUnconnected=off
  Omega : Outport  Port=2  Unit=rad/s  VectorParamsAs1DForOutWhenUnconnected=off
  Fx : Outport  Port=3  Unit=N  VectorParamsAs1DForOutWhenUnconnected=off
  Fy : Outport  Port=4  Unit=N  VectorParamsAs1DForOutWhenUnconnected=off
  Fz : Outport  Port=5  Unit=N  VectorParamsAs1DForOutWhenUnconnected=off
  Mx : Outport  Port=6  Unit=N*m  VectorParamsAs1DForOutWhenUnconnected=off
  My : Outport  Port=7  Unit=N*m  VectorParamsAs1DForOutWhenUnconnected=off
  Mz : Outport  Port=8  Unit=N*m  VectorParamsAs1DForOutWhenUnconnected=off
  wires:
  RadialDeflct/1 -> Signal Specification10/1
  Signal Specification10/1 -> Bus Creator/27  "RadialDeflct"
  Signal Specification9/1 -> Bus Creator/26  "RL"
  RL/1 -> Signal Specification9/1
  Signal Specification8/1 -> Bus Creator/25  "WhlTrq"
  WhlTrq/1 -> Signal Specification8/1
  Signal Specification3/1 -> Bus Creator/20  "z"
  a/1 -> Signal Specification23/1
  Alpha/1 -> Signal Specification2/1
  Signal Specification4/1 -> Bus Creator/21  "zdot"
  Signal Specification21/1 -> Bus Creator/2, Omega/1  "Omega"
  Fext/1 -> Signal Specification6/1
  Signal Specification15/1 -> Bus Creator/8, Mz/1  "Mz"
  Signal Specification/1 -> Bus Creator/11  "Re"
  Bus Creator/1 -> Info/1
  Signal Specification17/1 -> Mx/1, Bus Creator/6  "Mx"
  MOver/1 -> Signal Specification17/1
  Signal Specification1/1 -> Bus Creator/12  "Kappa"
  FLong/1 -> Signal Specification20/1
  Signal Specification19/1 -> Bus Creator/4, Fy/1  "Fy"
  Signal Specification16/1 -> Bus Creator/7, My/1  "My"
  omega/1 -> Signal Specification21/1
  Signal Specification2/1 -> Bus Creator/13  "Alpha"
  Signal Specification20/1 -> Bus Creator/3, Fx/1  "Fx"
  Signal Specification23/1 -> Bus Creator/14  "a"
  Signal Specification22/1 -> Bus Creator/15  "b"
  GndFz/1 -> Signal Specification18/1
  MAlign/1 -> Signal Specification15/1
  Flat/1 -> Signal Specification19/1
  b/1 -> Signal Specification22/1
  Re/1 -> Signal Specification/1
  zdot/1 -> Signal Specification4/1
  z/1 -> Signal Specification3/1
  MRoll/1 -> Signal Specification16/1
  Kappa/1 -> Signal Specification1/1
  BrkTrq/1 -> Signal Specification5/1
  AxlTrq/1 -> Bus Creator/1  "AxlTrq"
  Vx/1 -> Bus Creator/9  "Vx"
  Vy/1 -> Bus Creator/10  "Vy"
  Gamma/1 -> Bus Creator/16  "Gamma"
  psidot/1 -> Bus Creator/17  "psidot"
  Signal Specification5/1 -> Bus Creator/18  "BrkTrq"
  BrkPrs/1 -> Bus Creator/19  "BrkPrs"
  Signal Specification18/1 -> Bus Creator/23  "GndFz"
  Gnd/1 -> Signal Specification7/1
  Prs/1 -> Bus Creator/24  "Prs"
  Signal Specification6/1 -> Bus Creator/5, Fz/1  "Fz"
  Signal Specification7/1 -> Bus Creator/22  "Gnd"

== system Phase1_Mark2/Longitudinal Wheels 4DOF/Tires/Fiala/Fiala Tire/Fiala ==
  Omega : Inport
  GndFz : Inport  Port=2
  Vx : Inport  Port=3
  Vy : Inport  Port=4
  Gamma : Inport  Port=5
  psidot : Inport  Port=6
  Prs : Inport  Port=7
  ScaleFctrs : Inport  Port=8
  Tamb : Inport  Port=9
  RadialDeflct : Inport  Port=10
  MATLAB Function : MATLAB Function  TreatAsAtomicUnit=on
  Rolling : Subsystem  Variant=on  VariantControlMode=label  VariantControl=Variant1  LabelModeActiveChoice=Simple
  Slip : Subsystem
  Slip Angle : Subsystem
  Terminator9 : Terminator
  Fx : Outport  VectorParamsAs1DForOutWhenUnconnected=off
  Fy : Outport  Port=2  VectorParamsAs1DForOutWhenUnconnected=off
  Mx : Outport  Port=3  VectorParamsAs1DForOutWhenUnconnected=off
  My : Outport  Port=4  VectorParamsAs1DForOutWhenUnconnected=off
  Mz : Outport  Port=5  VectorParamsAs1DForOutWhenUnconnected=off
  Re : Outport  Port=6  VectorParamsAs1DForOutWhenUnconnected=off
  Kappa : Outport  Port=7  VectorParamsAs1DForOutWhenUnconnected=off
  Alpha : Outport  Port=8  VectorParamsAs1DForOutWhenUnconnected=off
  wires:
  MATLAB Function/1(Fx) -> Fx/1, Rolling/5(Fx)
  Prs/1 -> Rolling/7(Prs), MATLAB Function/5(prs)
  Omega/1 -> Slip/1(Omega), Rolling/1("Omega ")
  GndFz/1 -> Rolling/2("Fz "), MATLAB Function/6(Fz)
  Gamma/1 -> Rolling/6(gamma), MATLAB Function/3(gamma)
  MATLAB Function/5(Re) -> Slip/3(Re), Re/1, Rolling/3(Re)
  Vx/1 -> Slip Angle/1(Vx), Slip/2(Vx), Rolling/4(Vx), MATLAB Function/1(Vx)
  psidot/1 -> MATLAB Function/4(psidot)
  Slip Angle/2(Alpha) -> MATLAB Function/10(alpha), Alpha/1
  RadialDeflct/1 -> MATLAB Function/7(rhoz)
  Slip/1(Kappa) -> Kappa/1, MATLAB Function/9(kappa)
  Tamb/1 -> Rolling/8(Tamb)
  MATLAB Function/2(Fy) -> Fy/1
  Vy/1 -> Slip Angle/2(Vy), MATLAB Function/2(Vy)
  Slip Angle/1(tanalpha) -> Terminator9/1
  MATLAB Function/3(Mx) -> Mx/1
  Rolling/1(" My") -> My/1
  ScaleFctrs/1 -> MATLAB Function/8(ScaleFctr)
  MATLAB Function/4(Mz) -> Mz/1

== system Phase1_Mark2/Longitudinal Wheels 4DOF/Tires/Fiala/Fiala Tire/My Relaxation ==
  Omega : Inport
  Vx : Inport  Port=2
  My : Inport  Port=3
  Re : Inport  Port=4
  sig_x : Inport  Port=5
  Abs : Abs  ZeroCross=off  SaturateOnIntegerOverflow=off
  Add : Sum  Inputs=+-
  Add1 : Sum  Inputs=+-
  Integrator : Integrator  UpperSaturationLimit=10e3  LowerSaturationLimit=-10e3  AbsoluteTolerance=1e-2  ZeroCross=off
  Product1 : Product  Inputs=**
  Product2 : Product  Inputs=**
  Product3 : Product  Inputs=*/
  Saturation : Saturate  UpperLimit=inf  LowerLimit=MyRelFreqLwrLim  ZeroCross=off
  Saturation1 : Saturate  UpperLimit=inf  LowerLimit=1e-2  ZeroCross=off
  y : Outport  VectorParamsAs1DForOutWhenUnconnected=off
  wires:
  Product3/1 -> Saturation/1
  Saturation/1 -> Product1/1
  Product2/1 -> Add1/2
  Vx/1 -> Add1/1
  Re/1 -> Product2/2
  Omega/1 -> Product2/1
  My/1 -> Add/1
  Product1/1 -> Integrator/1
  Add/1 -> Product1/2
  Add1/1 -> Abs/1
  sig_x/1 -> Saturation1/1
  Saturation1/1 -> Product3/2
  Integrator/1 -> y/1, Add/2
  Abs/1 -> Product3/1

== system Phase1_Mark2/Longitudinal Wheels 4DOF/Tires/Fiala/Fiala Tire/Vertical DOF ==
  "GroundInput " : Inport
  "Fext " : Inport  Port=2
  rho : Inport  Port=3
  "GndFz " : Inport  Port=4
  Prs : Inport  Port=5
  External : Subsystem  VariantControl=vertType==3
  Mapped Vertical DOF : Subsystem  VariantControl=vertType==2
  None : Subsystem  VariantControl=vertType==1
  Vertical Wheel and Unsprung Mass Response : Subsystem  VariantControl=vertType==4  mask{m=MASS, bz=VERTICAL_DAMPING, zo=zo, zdoto=zdoto, g=GRAVITY, ReMax=UNLOADED_RADIUS}
      mask prompts: m "Unsprung mass [kg]"; bz "Vertical damping [N*m/s]"; zo "Initial deflection [m]"; zdoto "Initial velocity [m/s]"; g "Gravitational acceleration [m/s^2]"; ReMax "Maximum unloaded radius [m]:"
  RadialDeflct : Outport  VectorParamsAs1DForOutWhenUnconnected=off
  " z" : Outport  Port=2  VectorParamsAs1DForOutWhenUnconnected=off
  " zdot" : Outport  Port=3  VectorParamsAs1DForOutWhenUnconnected=off
  GndFz : Outport  Port=4  VectorParamsAs1DForOutWhenUnconnected=off

== system Phase1_Mark2/Longitudinal Wheels 4DOF/Tires/Fiala/Fiala Tire/Wheel Module ==
  BrkPrs : Inport
  AxlTrq : Inport  Port=2
  TireFdbk : Inport  Port=3
  RadialDeflct : Inport  Port=4
  Add1 : Sum  Inputs=--+
  Add2 : Sum  Inputs=-+
  Brakes : Subsystem  Variant=on  VariantControlMode=label  LabelModeActiveChoice=Disk  mask{aMode=aMode}
  Bus Selector1 : BusSelector  OutputSignals=My,Fx
  Clutch : Subsystem  Variant=on  VariantControlMode=label  VariantControl=Choice  LabelModeActiveChoice=0
  Constant9 : Constant  Value=UNLOADED_RADIUS
  Friction Model : Subsystem
  Product3 : Product  Inputs=**
  Reshape : Reshape
  Saturation : Saturate  UpperLimit=inf  LowerLimit=0  ZeroCross=off
  Terminator1 : Terminator
  Terminator3 : Terminator
  MyBrk : Outport  VectorParamsAs1DForOutWhenUnconnected=off
  Omega : Outport  Port=2  VectorParamsAs1DForOutWhenUnconnected=off
  wires:
  Reshape/1 -> Clutch/1(Tout)
  Product3/1 -> Add1/3
  AxlTrq/1 -> Add1/1
  RadialDeflct/1 -> Add2/1
  Friction Model/2(Tfmaxk) -> Clutch/3(Tfmaxk)
  Friction Model/1(Tfmaxs) -> Clutch/2(Tfmaxs)
  Add1/1 -> Reshape/1
  Clutch/3(Myb) -> Terminator1/1
  Clutch/2(Omegadot) -> Terminator3/1
  Clutch/1(Omega) -> Brakes/2(Omega), Omega/1
  Saturation/1 -> Product3/2
  Brakes/1(MyBrk) -> Friction Model/1(Brake torque), MyBrk/1
  Add2/1 -> Saturation/1
  Constant9/1 -> Add2/2
  BrkPrs/1 -> Brakes/1(BrkPrs)
  Bus Selector1/2 -> Product3/1  "<Fx>"
  Bus Selector1/1 -> Add1/2  "<My>"
  TireFdbk/1 -> Bus Selector1/1
